simulink model "Pointing_Cntrl_Act"  (R2013a)
settings: Solver=ode14x  StartTime=0.0  StopTime=500  FixedStep=0.01  RelTol=1e-3
values from neighbouring files (symbols this model uses):
  J1 = 4.2946e-2    (= 0.042946)    [RUNCODE_Pointing_CntrlACT.m]    (also in Satellite_Plant_Model.m = 0.000777537)
  J2 = 5.7648e-2    (= 0.057648)    [RUNCODE_Pointing_CntrlACT.m]    (also in Satellite_Plant_Model.m = 8.06522e-05)
  J3 = 1.9229e-2    (= 0.019229)    [RUNCODE_Pointing_CntrlACT.m]    (also in Satellite_Plant_Model.m = 0.0003439929)
  kq = 1    [Control_Block.m]    (also in RUNCODE_Pointing_CntrlACT.m)
  kw = 1    [Control_Block.m]    (also in RUNCODE_Pointing_CntrlACT.m)
  omega1_IC = 0    [RUNCODE_Pointing_CntrlACT.m]
  omega2_IC = 0    [RUNCODE_Pointing_CntrlACT.m]
  omega3_IC = 0    [RUNCODE_Pointing_CntrlACT.m]
  phi_des = 30    [RUNCODE_Pointing_CntrlACT.m]
  phi_dot_des = 0    [RUNCODE_Pointing_CntrlACT.m]
  psi_des = 90    [RUNCODE_Pointing_CntrlACT.m]
  psi_dot_des = 0    [RUNCODE_Pointing_CntrlACT.m]
  q1_IC = 0.1    [RUNCODE_Pointing_CntrlACT.m]
  q2_IC = 0.2    [RUNCODE_Pointing_CntrlACT.m]
  q3_IC = 0.3    [RUNCODE_Pointing_CntrlACT.m]
  q4_IC = 0.92736    [RUNCODE_Pointing_CntrlACT.m]
  theta_des = 120    [RUNCODE_Pointing_CntrlACT.m]
  theta_dot_des = 0    [RUNCODE_Pointing_CntrlACT.m]
  ts = 0.01    [RUNCODE_Pointing_CntrlACT.m]
libraries: dspmtrx3 x1
settings Model: Creator=Mike  LastModifiedBy=Mike

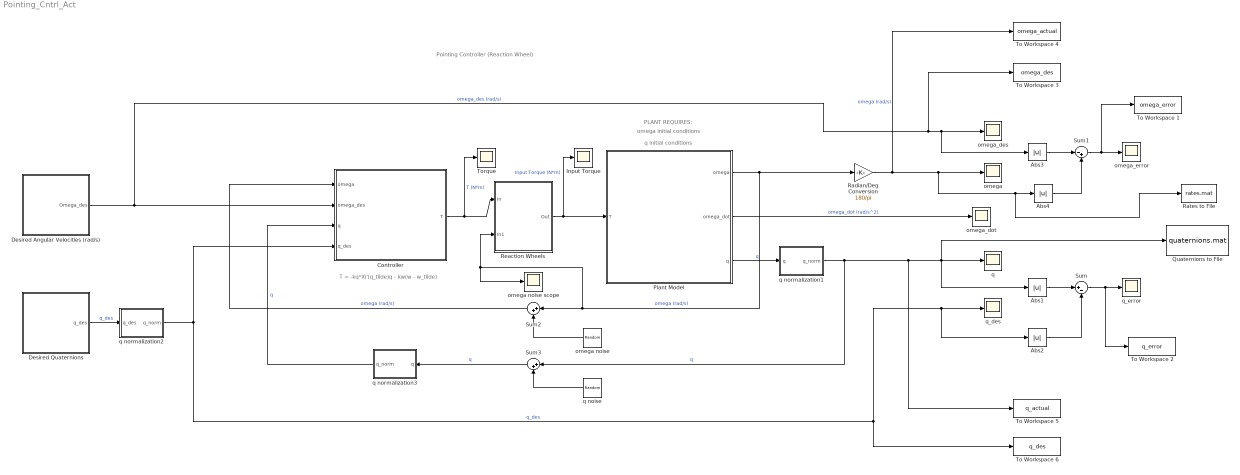
== system Pointing_Cntrl_Act ==
  note: T = -kq*Xi'(q_tilde)q - kw(w - w_tilde)
  note: omega initial conditions
  note: PLANT REQUIRES:
  note: q initial conditions
  note: Pointing Controller (Reaction Wheel)
  " Controller" : Subsystem
  Abs{1..4} (4 alike) : Abs
  Desired Angular Velocities (rad/s) : Subsystem
  Desired Quaternions : Subsystem
  Input Torque : Scope
      settings: TimeRange=500  YMin=-0.0007  YMax=0.0007
  Plant Model : Subsystem
  Quaternions to File : ToFile  Filename=quaternions.mat  MatrixName=quat
  Radian/Deg Conversion : Gain  Gain=180/pi
  Rates to File : ToFile  Filename=rates.mat  MatrixName=omega
  "Reaction Wheels " : Subsystem
  Sum : Sum  Inputs=|+-
  Sum1 : Sum  Inputs=|-+
  Sum2 : Sum  Inputs=|++
  Sum3 : Sum  Inputs=|++
  To Workspace 1 : ToWorkspace  VariableName=omega_error  SampleTime=-1  SaveFormat=Timeseries
  To Workspace 2 : ToWorkspace  VariableName=q_error  SampleTime=-1  SaveFormat=Timeseries
  To Workspace 3 : ToWorkspace  VariableName=omega_des  SampleTime=-1  SaveFormat=Timeseries
  To Workspace 4 : ToWorkspace  VariableName=omega_actual  SampleTime=-1  SaveFormat=Timeseries
  To Workspace 5 : ToWorkspace  VariableName=q_actual  SampleTime=-1  SaveFormat=Timeseries
  To Workspace 6 : ToWorkspace  VariableName=q_des  SampleTime=-1  SaveFormat=Timeseries
  Torque : Scope
      settings: TimeRange=500  YMin=-0.25  YMax=0.275  SaveName=ScopeData5
  omega : Scope
      settings: TimeRange=500  YMin=-15  YMax=10  SaveName=ScopeData3
  omega noise : UniformRandomNumber  Minimum=-.035  Maximum=.035  SampleTime=ts
  omega noise scope : Scope
      settings: TimeRange=500  YMin=-0.55  YMax=0.3  SaveName=ScopeData10
  omega_des : Scope
      settings: YMin=-0.0025  YMax=0.0525  SaveName=ScopeData8
  omega_dot : Scope
      settings: TimeRange=3600  YMin=-0.0004  YMax=-2.5e-05
  omega_error : Scope
      settings: TimeRange=500  YMin=0  YMax=3.25  SaveName=ScopeData7
  q : Scope
      settings: TimeRange=500  YMin=0.225  YMax=0.775  SaveName=ScopeData2
  q noise : UniformRandomNumber  Minimum=-.006  Maximum=.006  SampleTime=ts
  q normalization1 : Subsystem
  q normalization2 : Subsystem
  q normalization3 : Subsystem
  q_des : Scope
      settings: TimeRange=3600  YMin=0.25  YMax=0.75  SaveName=ScopeData4
  q_error : Scope
      settings: TimeRange=3600  YMin=-2e-12  YMax=1e-12  SaveName=ScopeData6
  wires:
  Plant Model/2(omega_dot) -> omega_dot/1  "omega_dot (rad/s^2)"
  " Controller"/1(T) -> "Reaction Wheels "/1(In), Torque/1  "T (N*m)"
  Abs1/1 -> Sum/1
  Abs2/1 -> Sum/2
  Abs3/1 -> Sum1/1
  Abs4/1 -> Sum1/2
  "Reaction Wheels "/1(Out) -> Input Torque/1, Plant Model/1(T)  "Input Torque (N*m)"
  Plant Model/3(q) -> q normalization1/1(q)  "q"
  Desired Quaternions/1(q_des) -> q normalization2/1(q_des)  "q_des"
  Plant Model/1(omega) -> omega noise scope/1, "Reaction Wheels "/2(In1), Sum2/1, Radian/Deg Conversion/1  "omega (rad/s)"
  Sum3/1 -> q normalization3/1(q)  "q"
  q normalization3/1(q_norm) -> " Controller"/3(q)  "q"
  Sum2/1 -> " Controller"/1(omega)  "omega (rad/s)"
  omega noise/1 -> Sum2/2
  q noise/1 -> Sum3/2
  Radian/Deg Conversion/1 -> omega/1, Rates to File/1, Abs4/1, To Workspace 4/1  "omega (rad/s)"
  Desired Angular Velocities (rad/s)/1(Omega_des) -> " Controller"/2(omega_des), To Workspace 3/1, omega_des/1, Abs3/1  "omega_des (rad/s)"
  Sum1/1 -> To Workspace 1/1, omega_error/1
  Sum/1 -> To Workspace 2/1, q_error/1
  q normalization1/1(q_norm) -> Sum3/1, To Workspace 5/1, Quaternions to File/1, Abs1/1, q/1  "q"
  q normalization2/1(q_norm) -> To Workspace 6/1, Abs2/1, q_des/1, " Controller"/4(q_des)  "q_des"

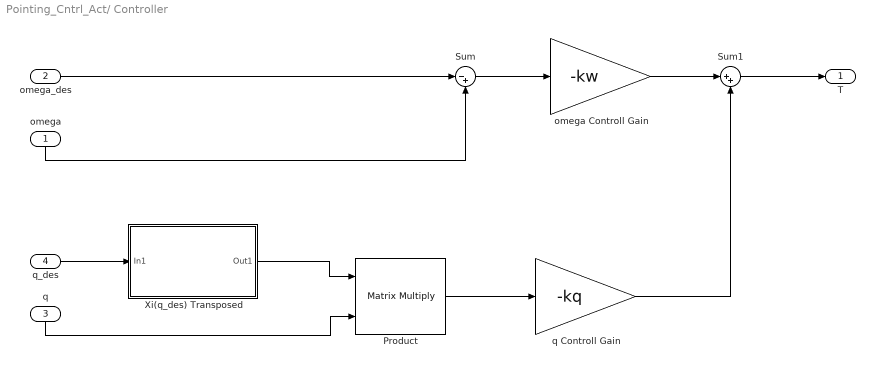
== system Pointing_Cntrl_Act/ Controller ==
  omega : Inport
  omega_des : Inport  Port=2
  q : Inport  Port=3
  q_des : Inport  Port=4
  Product : Product  Multiplication=Matrix(*)
  Sum : Sum  Inputs=|-+
  Sum1 : Sum  Inputs=|++
  Xi(q_des) Transposed : Subsystem
  omega Controll Gain : Gain  Gain=-kw
  q Controll Gain : Gain  Gain=-kq
  T : Outport
  wires:
  q_des/1 -> Xi(q_des) Transposed/1(In1)
  omega_des/1 -> Sum/1
  omega/1 -> Sum/2
  q/1 -> Product/2
  omega Controll Gain/1 -> Sum1/1
  Sum1/1 -> T/1
  Sum/1 -> omega Controll Gain/1
  Xi(q_des) Transposed/1(Out1) -> Product/1
  Product/1 -> q Controll Gain/1
  q Controll Gain/1 -> Sum1/2

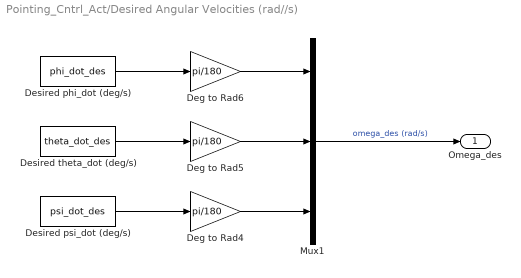
== system Pointing_Cntrl_Act/Desired Angular Velocities (rad//s) ==
  Deg to Rad4 : Gain  Gain=pi/180
  Deg to Rad5 : Gain  Gain=pi/180
  Deg to Rad6 : Gain  Gain=pi/180
  Desired phi_dot (deg/s) : Constant  Value=phi_dot_des
  Desired psi_dot (deg/s) : Constant  Value=psi_dot_des
  Desired theta_dot (deg/s) : Constant  Value=theta_dot_des
  Mux1 : Mux  Inputs=3
  Omega_des : Outport
  wires:
  Mux1/1 -> Omega_des/1  "omega_des (rad/s)"
  Deg to Rad4/1 -> Mux1/3
  Desired theta_dot (deg/s)/1 -> Deg to Rad5/1
  Desired psi_dot (deg/s)/1 -> Deg to Rad4/1
  Desired phi_dot (deg/s)/1 -> Deg to Rad6/1
  Deg to Rad6/1 -> Mux1/1
  Deg to Rad5/1 -> Mux1/2

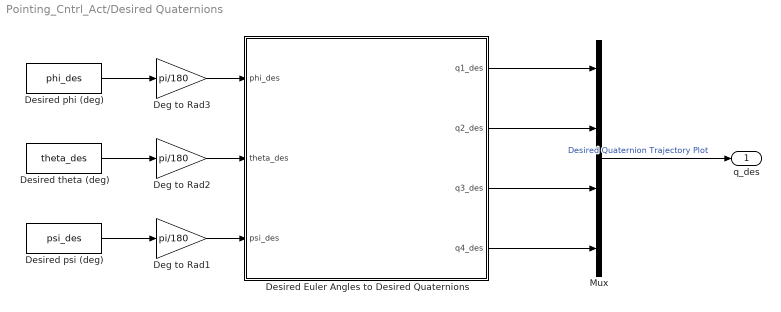
== system Pointing_Cntrl_Act/Desired Quaternions ==
  Deg to Rad1 : Gain  Gain=pi/180
  Deg to Rad2 : Gain  Gain=pi/180
  Deg to Rad3 : Gain  Gain=pi/180
  Desired Euler Angles to Desired Quaternions : MATLAB Function  TreatAsAtomicUnit=on
  Desired phi (deg) : Constant  Value=phi_des
  Desired psi (deg) : Constant  Value=psi_des
  Desired theta (deg) : Constant  Value=theta_des
  Mux : Mux
  q_des : Outport
  wires:
  Mux/1 -> q_des/1  "Desired Quaternion Trajectory Plot"
  Desired theta (deg)/1 -> Deg to Rad2/1
  Deg to Rad3/1 -> Desired Euler Angles to Desired Quaternions/1(phi_des)
  Desired Euler Angles to Desired Quaternions/2(q2_des) -> Mux/2
  Desired Euler Angles to Desired Quaternions/1(q1_des) -> Mux/1
  Deg to Rad1/1 -> Desired Euler Angles to Desired Quaternions/3(psi_des)
  Desired phi (deg)/1 -> Deg to Rad3/1
  Desired psi (deg)/1 -> Deg to Rad1/1
  Deg to Rad2/1 -> Desired Euler Angles to Desired Quaternions/2(theta_des)
  Desired Euler Angles to Desired Quaternions/3(q3_des) -> Mux/3
  Desired Euler Angles to Desired Quaternions/4(q4_des) -> Mux/4

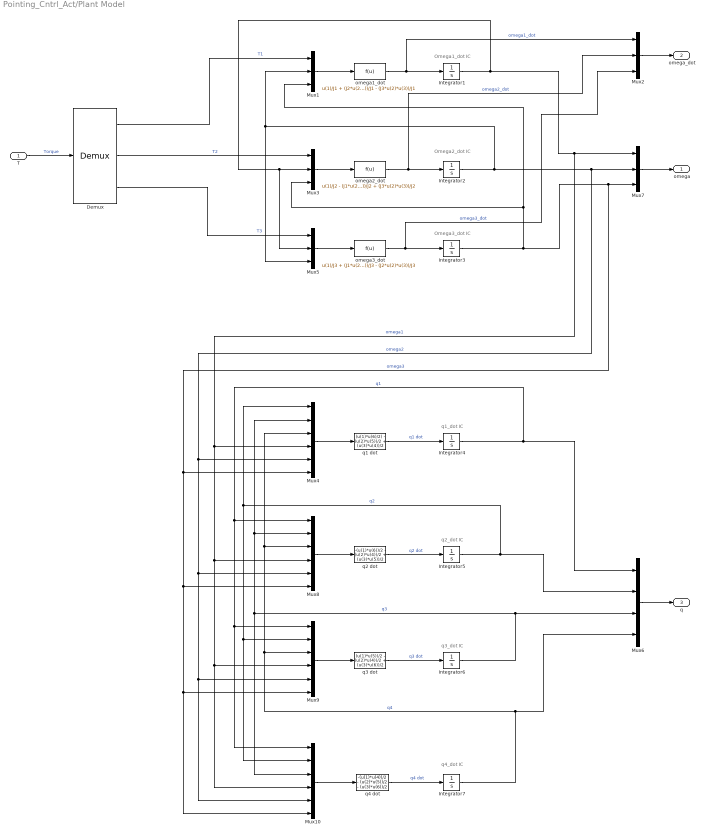
== system Pointing_Cntrl_Act/Plant Model ==
  note: Omega1_dot IC
  note: Omega2_dot IC
  note: Omega3_dot IC
  note: q1_dot IC
  note: q2_dot IC
  note: q3_dot IC
  note: q4_dot IC
  T : Inport
  Demux : Demux  Outputs=3
  Integrator1 : Integrator  InitialCondition=omega1_IC  AbsoluteTolerance=1e-3  ContinuousStateAttributes='omega1'
  Integrator2 : Integrator  InitialCondition=omega2_IC  AbsoluteTolerance=1e-3  ContinuousStateAttributes='omega2'
  Integrator3 : Integrator  InitialCondition=omega3_IC  AbsoluteTolerance=1e-3  ContinuousStateAttributes='omega3'
  Integrator4 : Integrator  InitialCondition=q1_IC  AbsoluteTolerance=1e-3  ContinuousStateAttributes='omega1'
  Integrator5 : Integrator  InitialCondition=q2_IC  AbsoluteTolerance=1e-3  ContinuousStateAttributes='omega1'
  Integrator6 : Integrator  InitialCondition=q3_IC  AbsoluteTolerance=1e-3  ContinuousStateAttributes='omega1'
  Integrator7 : Integrator  InitialCondition=q4_IC  AbsoluteTolerance=1e-3  ContinuousStateAttributes='omega1'
  Mux{1..3,5,7} (5 alike) : Mux  Inputs=3
  Mux{4,8..10} (4 alike) : Mux  Inputs=6
  Mux6 : Mux
  omega1_dot : Fcn  Expr=u(1)/J1 + (J2*u(2)*u(3))/J1 - (J3*u(2)*u(3))/J1
  omega2_dot : Fcn  Expr=u(1)/J2 - (J1*u(2)*u(3))/J2 + (J3*u(2)*u(3))/J2
  omega3_dot : Fcn  Expr=u(1)/J3 + (J1*u(2)*u(3))/J3 - (J2*u(2)*u(3))/J3
  q1 dot : Fcn  Expr=(u(1)*u(6)/2) - (u(2)*u(5))/2 + (u(3)*u(4))/2
  q2 dot : Fcn  Expr=-(u(1)*u(6))/2 - (u(2)*u(4))/2 + (u(3)*u(5))/2
  q3 dot : Fcn  Expr=(u(1)*u(5))/2 - (u(2)*u(4))/2 + (u(3)*u(6))/2
  q4 dot : Fcn  Expr=-(u(1)*u(4))/2 - (u(2)*u(5))/2 - (u(3)*u(6))/2
  omega : Outport
  omega_dot : Outport  Port=2
  q : Outport  Port=3
  wires:
  Demux/3 -> Mux5/1  "T3"
  T/1 -> Demux/1  "Torque"
  Mux7/1 -> omega/1
  Mux1/1 -> omega1_dot/1
  Integrator5/1 -> Mux9/2, Mux10/2, Mux4/1, Mux6/2  "q2"
  q3 dot/1 -> Integrator6/1  "q3 dot"
  Integrator6/1 -> Mux10/3, Mux8/2, Mux4/2, Mux6/3  "q3"
  Integrator7/1 -> Mux6/4, Mux9/3, Mux8/3, Mux4/3  "q4"
  omega3_dot/1 -> Mux2/3, Integrator3/1  "omega3_dot"
  Mux4/1 -> q1 dot/1
  omega2_dot/1 -> Mux2/2, Integrator2/1  "omega2_dot"
  q4 dot/1 -> Integrator7/1  "q4 dot"
  omega1_dot/1 -> Integrator1/1, Mux2/1  "omega1_dot"
  Mux5/1 -> omega3_dot/1
  q1 dot/1 -> Integrator4/1  "q1 dot"
  Mux8/1 -> q2 dot/1
  Integrator1/1 -> Mux7/1, Mux4/4, Mux8/4, Mux10/4, Mux9/4, Mux3/2, Mux5/2  "omega1"
  Integrator2/1 -> Mux7/2, Mux4/5, Mux8/5, Mux10/5, Mux9/5, Mux5/3, Mux1/2  "omega2"
  q2 dot/1 -> Integrator5/1  "q2 dot"
  Mux10/1 -> q4 dot/1
  Mux9/1 -> q3 dot/1
  Mux6/1 -> q/1
  Integrator4/1 -> Mux8/1, Mux9/1, Mux10/1, Mux6/1  "q1"
  Integrator3/1 -> Mux3/3, Mux1/3, Mux7/3, Mux4/6, Mux10/6, Mux9/6, Mux8/6  "omega3"
  Mux3/1 -> omega2_dot/1
  Demux/2 -> Mux3/1  "T2"
  Demux/1 -> Mux1/1  "T1"
  Mux2/1 -> omega_dot/1

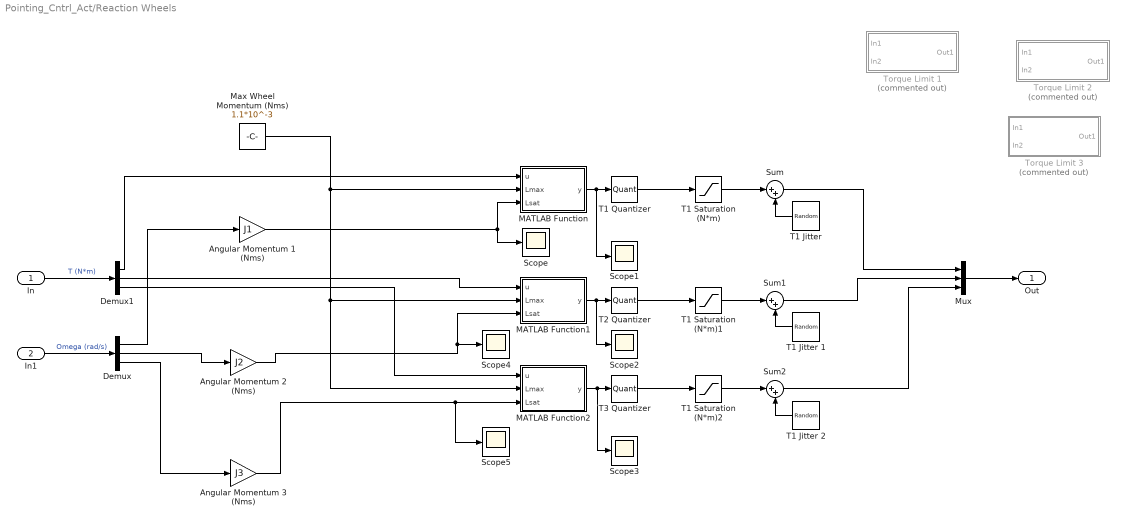
== system Pointing_Cntrl_Act/Reaction Wheels  ==
  In : Inport
  In1 : Inport  Port=2
  "Angular Momentum 1 (Nms) " : Gain  Gain=J1
  Angular Momentum 2 (Nms) : Gain  Gain=J2
  Angular Momentum 3 (Nms) : Gain  Gain=J3
  Demux : Demux  Outputs=3
  Demux1 : Demux  Outputs=3
  MATLAB Function : MATLAB Function  TreatAsAtomicUnit=on
  MATLAB Function1 : MATLAB Function  TreatAsAtomicUnit=on
  MATLAB Function2 : MATLAB Function  TreatAsAtomicUnit=on
  "Max Wheel Momentum (Nms) " : Constant  Value=1.1*10^-3
  Mux : Mux  Inputs=3
  Scope{,1..5} (6 alike) : Scope
      Scope settings: YMin=-0.0075  YMax=0.0175  SaveName=ScopeData11
      Scope1 settings: YMin=-7.5  YMax=0.5  SaveName=ScopeData12
      Scope2 settings: YMin=-0.0075  YMax=0.0175  SaveName=ScopeData13
      Scope3 settings: YMin=-0.0075  YMax=0.0175  SaveName=ScopeData14
      Scope4 settings: YMin=-0.0075  YMax=0.0175  SaveName=ScopeData15
      Scope5 settings: YMin=-0.0005  YMax=0.0005  SaveName=ScopeData16
  Sum : Sum  Inputs=|++
  Sum1 : Sum  Inputs=|++
  Sum2 : Sum  Inputs=|++
  "T1 Jitter " : UniformRandomNumber  Minimum=-0.0005*10^-3  Maximum=0.0005*10^-3  SampleTime=ts
  T1 Jitter 1 : UniformRandomNumber  Minimum=-0.0005*10^-3  Maximum=0.001*10^-3  SampleTime=ts
  T1 Jitter 2 : UniformRandomNumber  Minimum=-0.0005*10^-3  Maximum=0.001*10^-3  SampleTime=ts
  T1 Quantizer : Quantizer  QuantizationInterval=0.02*10^-3
  T1 Saturation (N*m) : Saturate  UpperLimit=0.635/1000  LowerLimit=-0.635/1000
  T1 Saturation (N*m)1 : Saturate  UpperLimit=0.635/1000  LowerLimit=-0.635/1000
  T1 Saturation (N*m)2 : Saturate  UpperLimit=0.635/1000  LowerLimit=-0.635/1000
  T2 Quantizer : Quantizer  QuantizationInterval=0.02*10^-3
  T3 Quantizer : Quantizer  QuantizationInterval=0.02*10^-3
  Torque Limit 1 : Subsystem  Commented=on  TreatAsAtomicUnit=on
  Torque Limit 2 : Subsystem  Commented=on  TreatAsAtomicUnit=on
  Torque Limit 3 : Subsystem  Commented=on  TreatAsAtomicUnit=on
  Out : Outport
  wires:
  In/1 -> Demux1/1  "T (N*m)"
  Demux1/2 -> MATLAB Function1/1(u)
  Demux1/1 -> MATLAB Function/1(u)
  Mux/1 -> Out/1
  In1/1 -> Demux/1  "Omega (rad/s)"
  Demux/1 -> "Angular Momentum 1 (Nms) "/1
  Demux/2 -> Angular Momentum 2 (Nms)/1
  Demux/3 -> Angular Momentum 3 (Nms)/1
  "Max Wheel Momentum (Nms) "/1 -> MATLAB Function/2(Lmax), MATLAB Function2/2(Lmax), MATLAB Function1/2(Lmax)
  Angular Momentum 2 (Nms)/1 -> Scope4/1, MATLAB Function1/3(Lsat)
  Angular Momentum 3 (Nms)/1 -> Scope5/1, MATLAB Function2/3(Lsat)
  T1 Quantizer/1 -> T1 Saturation (N*m)/1
  MATLAB Function/1(y) -> Scope1/1, T1 Quantizer/1
  T1 Saturation (N*m)/1 -> Sum/1
  Sum/1 -> Mux/1
  "T1 Jitter "/1 -> Sum/2
  MATLAB Function1/1(y) -> Scope2/1, T2 Quantizer/1
  T1 Saturation (N*m)1/1 -> Sum1/1
  T1 Jitter 1/1 -> Sum1/2
  T2 Quantizer/1 -> T1 Saturation (N*m)1/1
  Sum1/1 -> Mux/2
  T1 Saturation (N*m)2/1 -> Sum2/1
  T1 Jitter 2/1 -> Sum2/2
  T3 Quantizer/1 -> T1 Saturation (N*m)2/1
  Sum2/1 -> Mux/3
  MATLAB Function2/1(y) -> Scope3/1, T3 Quantizer/1
  Demux1/3 -> MATLAB Function2/1(u)
  "Angular Momentum 1 (Nms) "/1 -> MATLAB Function/3(Lsat), Scope/1

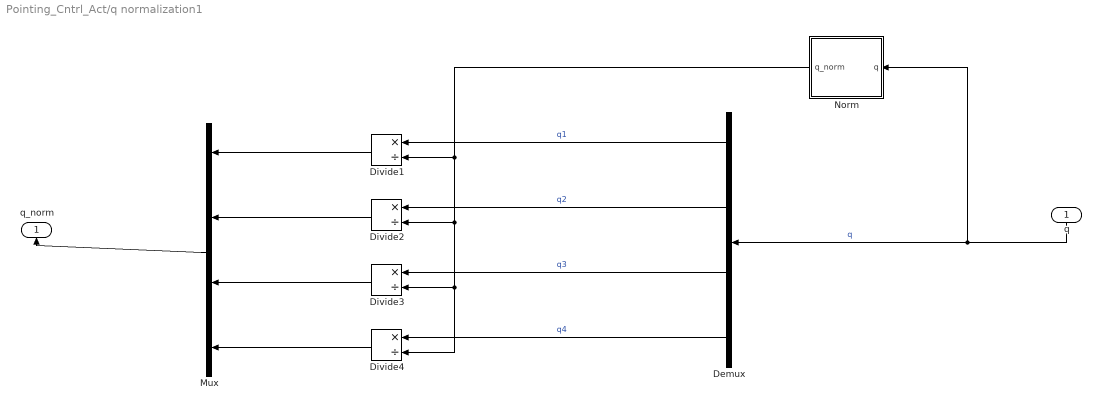
== system Pointing_Cntrl_Act/q normalization1 ==
  q : Inport
  Demux : Demux
  Divide{1..4} (4 alike) : Product  Inputs=*/
  Mux : Mux
  Norm : MATLAB Function  TreatAsAtomicUnit=on
  q_norm : Outport
  wires:
  Divide1/1 -> Mux/1
  Divide2/1 -> Mux/2
  Divide3/1 -> Mux/3
  Divide4/1 -> Mux/4
  Mux/1 -> q_norm/1
  Demux/2 -> Divide2/1  "q2"
  Demux/3 -> Divide3/1  "q3"
  Demux/4 -> Divide4/1  "q4"
  Demux/1 -> Divide1/1  "q1"
  Norm/1(q_norm) -> Divide1/2, Divide2/2, Divide3/2, Divide4/2
  q/1 -> Norm/1(q), Demux/1  "q"

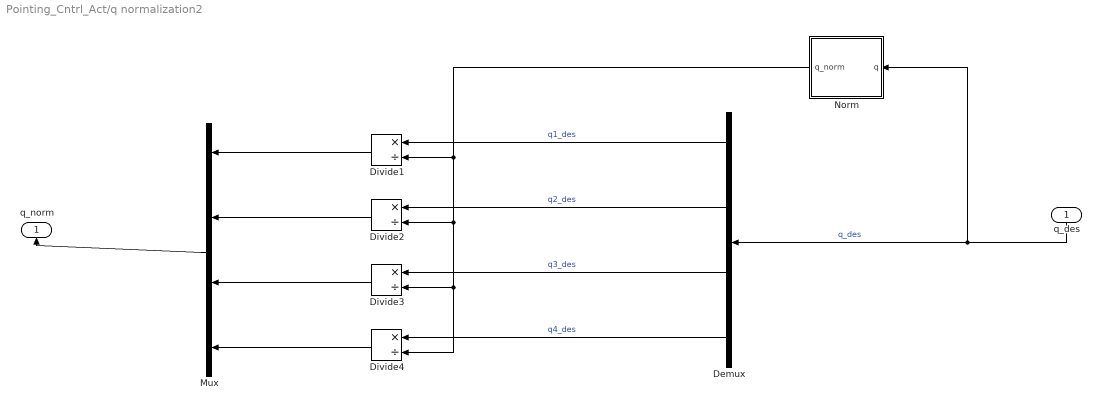
== system Pointing_Cntrl_Act/q normalization2 ==
  q_des : Inport
  Demux : Demux
  Divide{1..4} (4 alike) : Product  Inputs=*/
  Mux : Mux
  Norm : MATLAB Function  TreatAsAtomicUnit=on
  q_norm : Outport
  wires:
  Divide1/1 -> Mux/1
  Divide2/1 -> Mux/2
  Divide3/1 -> Mux/3
  Divide4/1 -> Mux/4
  Mux/1 -> q_norm/1
  Demux/2 -> Divide2/1  "q2_des"
  Demux/3 -> Divide3/1  "q3_des"
  Demux/4 -> Divide4/1  "q4_des"
  Demux/1 -> Divide1/1  "q1_des"
  Norm/1(q_norm) -> Divide1/2, Divide2/2, Divide3/2, Divide4/2
  q_des/1 -> Norm/1(q), Demux/1  "q_des"

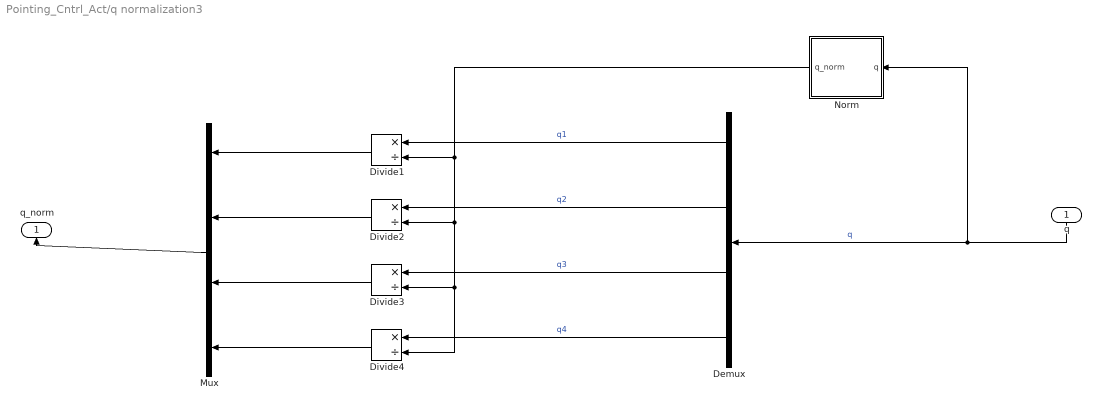
== system Pointing_Cntrl_Act/q normalization3 ==
  q : Inport
  Demux : Demux
  Divide{1..4} (4 alike) : Product  Inputs=*/
  Mux : Mux
  Norm : MATLAB Function  TreatAsAtomicUnit=on
  q_norm : Outport
  wires:
  Divide1/1 -> Mux/1
  Divide2/1 -> Mux/2
  Divide3/1 -> Mux/3
  Divide4/1 -> Mux/4
  Mux/1 -> q_norm/1
  Demux/2 -> Divide2/1  "q2"
  Demux/3 -> Divide3/1  "q3"
  Demux/4 -> Divide4/1  "q4"
  Demux/1 -> Divide1/1  "q1"
  Norm/1(q_norm) -> Divide1/2, Divide2/2, Divide3/2, Divide4/2
  q/1 -> Norm/1(q), Demux/1  "q"

== system Pointing_Cntrl_Act/ Controller/Xi(q_des) Transposed ==
  In1 : Inport
  Demux : Demux
  Transpose : dspmtrx3/Transpose  Hermitian=off  overflowFlag=off
  Xi_qtilde = Xi(q_des) : MATLAB Function  TreatAsAtomicUnit=on
  Out1 : Outport
  wires:
  In1/1 -> Demux/1
  Demux/4 -> Xi_qtilde = Xi(q_des)/4(q4_des)
  Demux/2 -> Xi_qtilde = Xi(q_des)/2(q2_des)
  Demux/1 -> Xi_qtilde = Xi(q_des)/1(q1_des)
  Transpose/1 -> Out1/1
  Xi_qtilde = Xi(q_des)/1(Xi_qtilde) -> Transpose/1
  Demux/3 -> Xi_qtilde = Xi(q_des)/3(q3_des)

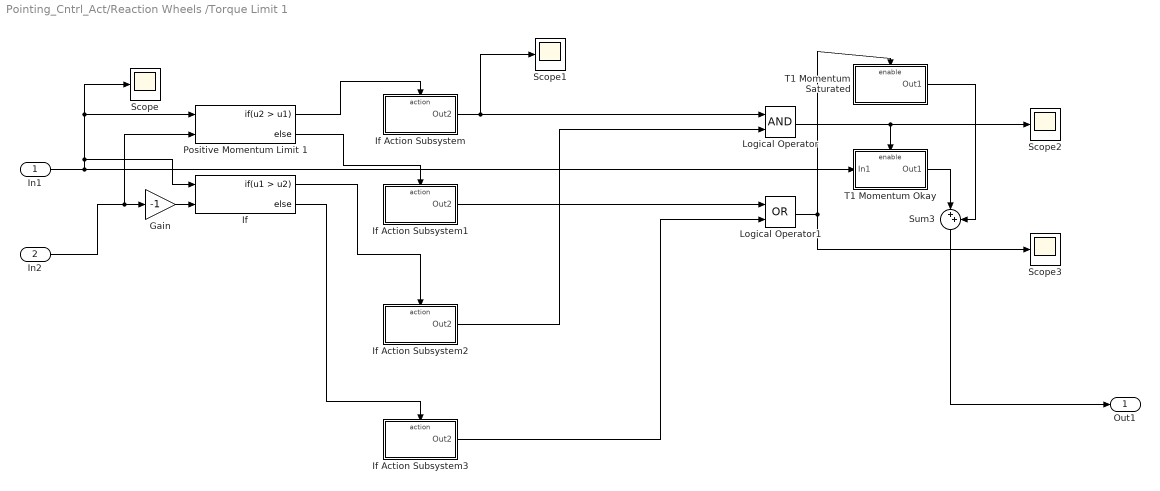
== system Pointing_Cntrl_Act/Reaction Wheels /Torque Limit 1 ==
  In1 : Inport
  In2 : Inport  Port=2
  Gain : Gain  Gain=-1
  If : If  NumInputs=2  IfExpression=u1 > u2
  If Action Subsystem : Subsystem  TreatAsAtomicUnit=on
  If Action Subsystem1 : Subsystem  TreatAsAtomicUnit=on
  If Action Subsystem2 : Subsystem  TreatAsAtomicUnit=on
  If Action Subsystem3 : Subsystem  TreatAsAtomicUnit=on
  Logical Operator : Logic  AllPortsSameDT=off  OutDataTypeStr=boolean
  Logical Operator1 : Logic  Operator=OR  AllPortsSameDT=off  OutDataTypeStr=boolean
  Positive Momentum Limit 1 : If  NumInputs=2  IfExpression=u2 > u1
  Scope{,1..3} (4 alike) : Scope
      Scope settings: YMin=-1.5  YMax=8  SaveName=ScopeData17
      Scope1 settings: YMin=-1.5  YMax=8  SaveName=ScopeData18
      Scope2 settings: YMin=-1.5  YMax=8  SaveName=ScopeData19
      Scope3 settings: YMin=-1.5  YMax=8  SaveName=ScopeData20
  Sum3 : Sum  Inputs=|++
  T1 Momentum Okay : Subsystem  TreatAsAtomicUnit=on
  "T1 Momentum Saturated " : Subsystem  TreatAsAtomicUnit=on
  Out1 : Outport
  wires:
  In1/1 -> T1 Momentum Okay/1(In1), Scope/1, Positive Momentum Limit 1/1, If/1
  In2/1 -> Positive Momentum Limit 1/2, Gain/1
  T1 Momentum Okay/1(Out1) -> Sum3/1
  Sum3/1 -> Out1/1
  "T1 Momentum Saturated "/1(Out1) -> Sum3/2
  Gain/1 -> If/2
  Logical Operator/1 -> Scope2/1, T1 Momentum Okay/Enable
  Logical Operator1/1 -> "T1 Momentum Saturated "/Enable, Scope3/1
  Positive Momentum Limit 1/1 -> If Action Subsystem/Action
  If/2 -> If Action Subsystem3/Action
  Positive Momentum Limit 1/2 -> If Action Subsystem1/Action
  If/1 -> If Action Subsystem2/Action
  If Action Subsystem/1(Out2) -> Scope1/1, Logical Operator/1
  If Action Subsystem2/1(Out2) -> Logical Operator/2
  If Action Subsystem1/1(Out2) -> Logical Operator1/1
  If Action Subsystem3/1(Out2) -> Logical Operator1/2

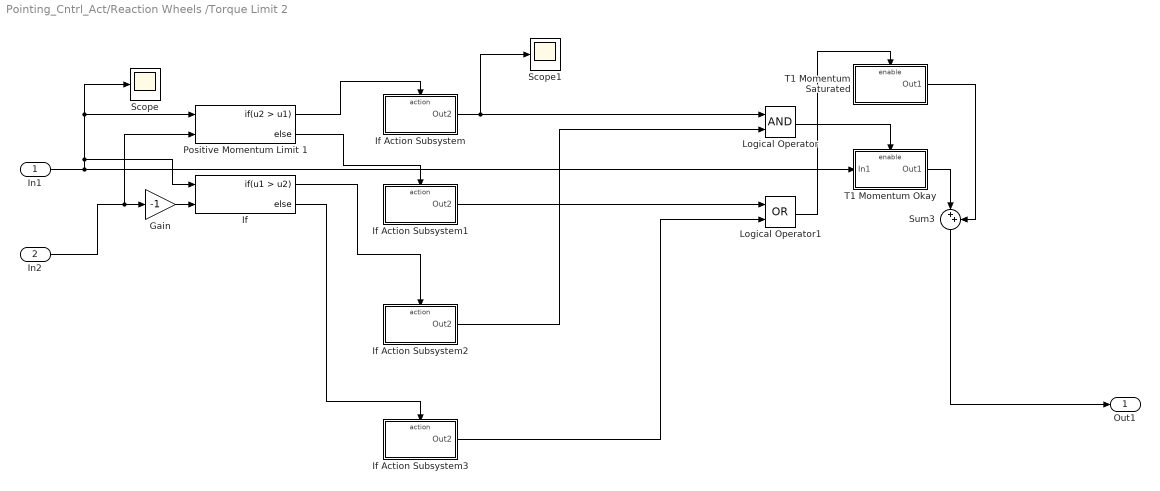
== system Pointing_Cntrl_Act/Reaction Wheels /Torque Limit 2 ==
  In1 : Inport
  In2 : Inport  Port=2
  Gain : Gain  Gain=-1
  If : If  NumInputs=2  IfExpression=u1 > u2
  If Action Subsystem : Subsystem  TreatAsAtomicUnit=on
  If Action Subsystem1 : Subsystem  TreatAsAtomicUnit=on
  If Action Subsystem2 : Subsystem  TreatAsAtomicUnit=on
  If Action Subsystem3 : Subsystem  TreatAsAtomicUnit=on
  Logical Operator : Logic  AllPortsSameDT=off  OutDataTypeStr=boolean
  Logical Operator1 : Logic  Operator=OR  AllPortsSameDT=off  OutDataTypeStr=boolean
  Positive Momentum Limit 1 : If  NumInputs=2  IfExpression=u2 > u1
  Scope : Scope
      settings: YMin=-1.5  YMax=8  SaveName=ScopeData17
  Scope1 : Scope
      settings: YMin=-1.5  YMax=8  SaveName=ScopeData18
  Sum3 : Sum  Inputs=|++
  T1 Momentum Okay : Subsystem  TreatAsAtomicUnit=on
  "T1 Momentum Saturated " : Subsystem  TreatAsAtomicUnit=on
  Out1 : Outport
  wires:
  In1/1 -> T1 Momentum Okay/1(In1), Scope/1, Positive Momentum Limit 1/1, If/1
  In2/1 -> Positive Momentum Limit 1/2, Gain/1
  T1 Momentum Okay/1(Out1) -> Sum3/1
  Sum3/1 -> Out1/1
  "T1 Momentum Saturated "/1(Out1) -> Sum3/2
  Gain/1 -> If/2
  Logical Operator/1 -> T1 Momentum Okay/Enable
  Logical Operator1/1 -> "T1 Momentum Saturated "/Enable
  Positive Momentum Limit 1/1 -> If Action Subsystem/Action
  If/2 -> If Action Subsystem3/Action
  Positive Momentum Limit 1/2 -> If Action Subsystem1/Action
  If/1 -> If Action Subsystem2/Action
  If Action Subsystem/1(Out2) -> Scope1/1, Logical Operator/1
  If Action Subsystem2/1(Out2) -> Logical Operator/2
  If Action Subsystem1/1(Out2) -> Logical Operator1/1
  If Action Subsystem3/1(Out2) -> Logical Operator1/2

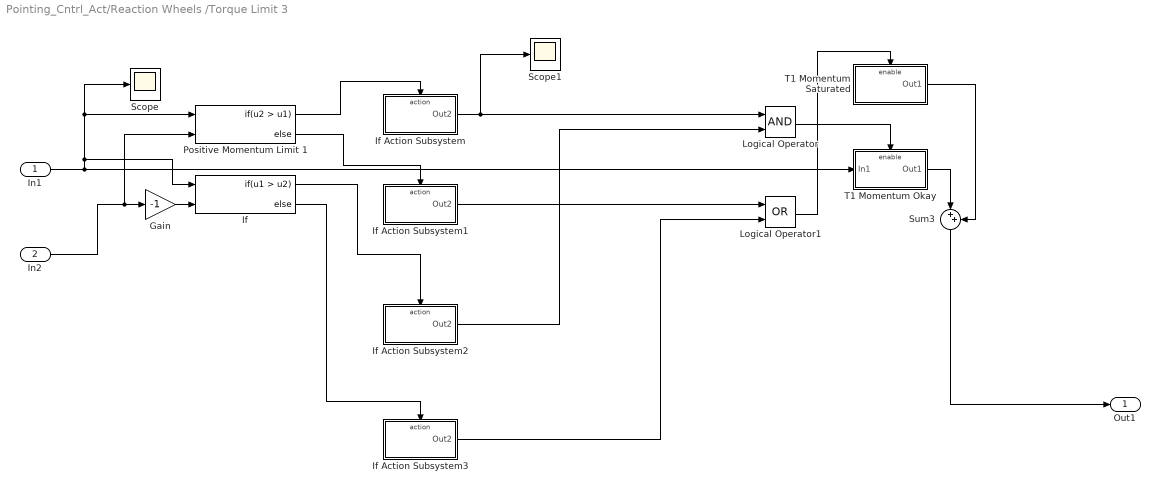
== system Pointing_Cntrl_Act/Reaction Wheels /Torque Limit 3 ==
  In1 : Inport
  In2 : Inport  Port=2
  Gain : Gain  Gain=-1
  If : If  NumInputs=2  IfExpression=u1 > u2
  If Action Subsystem : Subsystem  TreatAsAtomicUnit=on
  If Action Subsystem1 : Subsystem  TreatAsAtomicUnit=on
  If Action Subsystem2 : Subsystem  TreatAsAtomicUnit=on
  If Action Subsystem3 : Subsystem  TreatAsAtomicUnit=on
  Logical Operator : Logic  AllPortsSameDT=off  OutDataTypeStr=boolean
  Logical Operator1 : Logic  Operator=OR  AllPortsSameDT=off  OutDataTypeStr=boolean
  Positive Momentum Limit 1 : If  NumInputs=2  IfExpression=u2 > u1
  Scope : Scope
      settings: YMin=-1.5  YMax=8  SaveName=ScopeData17
  Scope1 : Scope
      settings: YMin=-1.5  YMax=8  SaveName=ScopeData18
  Sum3 : Sum  Inputs=|++
  T1 Momentum Okay : Subsystem  TreatAsAtomicUnit=on
  "T1 Momentum Saturated " : Subsystem  TreatAsAtomicUnit=on
  Out1 : Outport
  wires:
  In1/1 -> T1 Momentum Okay/1(In1), Scope/1, Positive Momentum Limit 1/1, If/1
  In2/1 -> Positive Momentum Limit 1/2, Gain/1
  T1 Momentum Okay/1(Out1) -> Sum3/1
  Sum3/1 -> Out1/1
  "T1 Momentum Saturated "/1(Out1) -> Sum3/2
  Gain/1 -> If/2
  Logical Operator/1 -> T1 Momentum Okay/Enable
  Logical Operator1/1 -> "T1 Momentum Saturated "/Enable
  Positive Momentum Limit 1/1 -> If Action Subsystem/Action
  If/2 -> If Action Subsystem3/Action
  Positive Momentum Limit 1/2 -> If Action Subsystem1/Action
  If/1 -> If Action Subsystem2/Action
  If Action Subsystem/1(Out2) -> Scope1/1, Logical Operator/1
  If Action Subsystem2/1(Out2) -> Logical Operator/2
  If Action Subsystem1/1(Out2) -> Logical Operator1/1
  If Action Subsystem3/1(Out2) -> Logical Operator1/2

== system Pointing_Cntrl_Act/Reaction Wheels /Torque Limit 1/If Action Subsystem ==
  Action Port : ActionPort  InitializeStates=reset
  Constant : Constant  Value=true  OutDataTypeStr=boolean
  Out2 : Outport  OutDataTypeStr=boolean  OutputWhenDisabled=reset  InitialOutput=[false]
  wires:
  Constant/1 -> Out2/1

== system Pointing_Cntrl_Act/Reaction Wheels /Torque Limit 1/If Action Subsystem1 ==
  Action Port : ActionPort  InitializeStates=reset
  Constant : Constant  Value=true  OutDataTypeStr=boolean
  Out2 : Outport  OutDataTypeStr=boolean  OutputWhenDisabled=reset  InitialOutput=[false]
  wires:
  Constant/1 -> Out2/1

== system Pointing_Cntrl_Act/Reaction Wheels /Torque Limit 1/If Action Subsystem2 ==
  Action Port : ActionPort  InitializeStates=reset
  Constant : Constant  Value=true  OutDataTypeStr=boolean
  Out2 : Outport  OutDataTypeStr=boolean  OutputWhenDisabled=reset  InitialOutput=[false]
  wires:
  Constant/1 -> Out2/1

== system Pointing_Cntrl_Act/Reaction Wheels /Torque Limit 1/If Action Subsystem3 ==
  Action Port : ActionPort  InitializeStates=reset
  Constant : Constant  Value=true  OutDataTypeStr=boolean
  Out2 : Outport  OutDataTypeStr=boolean  OutputWhenDisabled=reset  InitialOutput=[false]
  wires:
  Constant/1 -> Out2/1

== system Pointing_Cntrl_Act/Reaction Wheels /Torque Limit 1/T1 Momentum Okay ==
  In1 : Inport
  Enable : EnablePort  StatesWhenEnabling=reset
  Sum : Sum  Inputs=|++
  "T1 Jitter " : UniformRandomNumber  Minimum=-0.005  Maximum=0.005  SampleTime=ts
  T1 Saturation (N*m) : Saturate  UpperLimit=0.635/1000  LowerLimit=-0.635/1000
  Out1 : Outport  InitialOutput=[0]
  wires:
  T1 Saturation (N*m)/1 -> Sum/1
  "T1 Jitter "/1 -> Sum/2
  Sum/1 -> Out1/1
  In1/1 -> T1 Saturation (N*m)/1

== system Pointing_Cntrl_Act/Reaction Wheels /Torque Limit 1/T1 Momentum Saturated  ==
  Enable : EnablePort  StatesWhenEnabling=reset
  "T1 Jitter " : UniformRandomNumber  Minimum=-0.005  Maximum=0.005  SampleTime=ts
  Out1 : Outport  InitialOutput=[0]
  wires:
  "T1 Jitter "/1 -> Out1/1

== system Pointing_Cntrl_Act/Reaction Wheels /Torque Limit 2/If Action Subsystem ==
  Action Port : ActionPort  InitializeStates=reset
  Constant : Constant  Value=true  OutDataTypeStr=boolean
  Out2 : Outport  OutDataTypeStr=boolean  OutputWhenDisabled=reset  InitialOutput=[false]
  wires:
  Constant/1 -> Out2/1

== system Pointing_Cntrl_Act/Reaction Wheels /Torque Limit 2/If Action Subsystem1 ==
  Action Port : ActionPort  InitializeStates=reset
  Constant : Constant  Value=true  OutDataTypeStr=boolean
  Out2 : Outport  OutDataTypeStr=boolean  OutputWhenDisabled=reset  InitialOutput=[false]
  wires:
  Constant/1 -> Out2/1

== system Pointing_Cntrl_Act/Reaction Wheels /Torque Limit 2/If Action Subsystem2 ==
  Action Port : ActionPort  InitializeStates=reset
  Constant : Constant  Value=true  OutDataTypeStr=boolean
  Out2 : Outport  OutDataTypeStr=boolean  OutputWhenDisabled=reset  InitialOutput=[false]
  wires:
  Constant/1 -> Out2/1

== system Pointing_Cntrl_Act/Reaction Wheels /Torque Limit 2/If Action Subsystem3 ==
  Action Port : ActionPort  InitializeStates=reset
  Constant : Constant  Value=true  OutDataTypeStr=boolean
  Out2 : Outport  OutDataTypeStr=boolean  OutputWhenDisabled=reset  InitialOutput=[false]
  wires:
  Constant/1 -> Out2/1

== system Pointing_Cntrl_Act/Reaction Wheels /Torque Limit 2/T1 Momentum Okay ==
  In1 : Inport
  Enable : EnablePort  StatesWhenEnabling=reset
  Sum : Sum  Inputs=|++
  "T1 Jitter " : UniformRandomNumber  Minimum=-0.005  Maximum=0.005  SampleTime=ts
  T1 Saturation (N*m) : Saturate  UpperLimit=0.635/1000  LowerLimit=-0.635/1000
  Out1 : Outport  InitialOutput=[0]
  wires:
  T1 Saturation (N*m)/1 -> Sum/1
  "T1 Jitter "/1 -> Sum/2
  Sum/1 -> Out1/1
  In1/1 -> T1 Saturation (N*m)/1

== system Pointing_Cntrl_Act/Reaction Wheels /Torque Limit 2/T1 Momentum Saturated  ==
  Enable : EnablePort  StatesWhenEnabling=reset
  "T1 Jitter " : UniformRandomNumber  Minimum=-0.005  Maximum=0.005  SampleTime=ts
  Out1 : Outport  InitialOutput=[0]
  wires:
  "T1 Jitter "/1 -> Out1/1

== system Pointing_Cntrl_Act/Reaction Wheels /Torque Limit 3/If Action Subsystem ==
  Action Port : ActionPort  InitializeStates=reset
  Constant : Constant  Value=true  OutDataTypeStr=boolean
  Out2 : Outport  OutDataTypeStr=boolean  OutputWhenDisabled=reset  InitialOutput=[false]
  wires:
  Constant/1 -> Out2/1

== system Pointing_Cntrl_Act/Reaction Wheels /Torque Limit 3/If Action Subsystem1 ==
  Action Port : ActionPort  InitializeStates=reset
  Constant : Constant  Value=true  OutDataTypeStr=boolean
  Out2 : Outport  OutDataTypeStr=boolean  OutputWhenDisabled=reset  InitialOutput=[false]
  wires:
  Constant/1 -> Out2/1

== system Pointing_Cntrl_Act/Reaction Wheels /Torque Limit 3/If Action Subsystem2 ==
  Action Port : ActionPort  InitializeStates=reset
  Constant : Constant  Value=true  OutDataTypeStr=boolean
  Out2 : Outport  OutDataTypeStr=boolean  OutputWhenDisabled=reset  InitialOutput=[false]
  wires:
  Constant/1 -> Out2/1

== system Pointing_Cntrl_Act/Reaction Wheels /Torque Limit 3/If Action Subsystem3 ==
  Action Port : ActionPort  InitializeStates=reset
  Constant : Constant  Value=true  OutDataTypeStr=boolean
  Out2 : Outport  OutDataTypeStr=boolean  OutputWhenDisabled=reset  InitialOutput=[false]
  wires:
  Constant/1 -> Out2/1

== system Pointing_Cntrl_Act/Reaction Wheels /Torque Limit 3/T1 Momentum Okay ==
  In1 : Inport
  Enable : EnablePort  StatesWhenEnabling=reset
  Sum : Sum  Inputs=|++
  "T1 Jitter " : UniformRandomNumber  Minimum=-0.005  Maximum=0.005  SampleTime=ts
  T1 Saturation (N*m) : Saturate  UpperLimit=0.635/1000  LowerLimit=-0.635/1000
  Out1 : Outport  InitialOutput=[0]
  wires:
  T1 Saturation (N*m)/1 -> Sum/1
  "T1 Jitter "/1 -> Sum/2
  Sum/1 -> Out1/1
  In1/1 -> T1 Saturation (N*m)/1

== system Pointing_Cntrl_Act/Reaction Wheels /Torque Limit 3/T1 Momentum Saturated  ==
  Enable : EnablePort  StatesWhenEnabling=reset
  "T1 Jitter " : UniformRandomNumber  Minimum=-0.005  Maximum=0.005  SampleTime=ts
  Out1 : Outport  InitialOutput=[0]
  wires:
  "T1 Jitter "/1 -> Out1/1

== matlab function Pointing_Cntrl_Act/Reaction Wheels /MATLAB Function ==
  data: u input; y output; Lmax input; Lsat input
function y = fcn(u,Lmax,Lsat)
%#codegen

if u >= 0
    Llim = Lmax - Lsat;
    if Llim < 0
        y = 0;
    else
        y = min (Llim,u);
    end
else
    Llim = -Lmax - Lsat;
    if Llim > 0
        y = 0;
    else
        y = max(Llim,u);
    end
end

== matlab function Pointing_Cntrl_Act/ Controller/Xi(q_des) Transposed/Xi_qtilde = Xi(q_des) ==
  data: q1_des input; Xi_qtilde output; q2_des input; q3_des input; q4_des input
function Xi_qtilde = fcn(q1_des,q2_des,q3_des,q4_des)
Xi_qtilde=[q4_des  -q3_des   q2_des;
           q3_des   q4_des  -q1_des;
          -q2_des   q1_des   q4_des;
          -q1_des  -q2_des  -q3_des];

== matlab function Pointing_Cntrl_Act/q normalization2/Norm ==
  data: q input; q_norm output
function q_norm = fcn(q)

q_norm = norm(q);

== matlab function Pointing_Cntrl_Act/Reaction Wheels /MATLAB Function1 ==
  data: u input; y output; Lmax input; Lsat input
function y = fcn(u,Lmax,Lsat)
%#codegen

if u >= 0
    Llim = Lmax - Lsat;
    if Llim < 0
        y = 0;
    else
        y = min (Llim,u);
    end
else
    Llim = -Lmax - Lsat;
    if Llim > 0
        y = 0;
    else
        y = max(Llim,u);
    end
end

== matlab function Pointing_Cntrl_Act/q normalization3/Norm ==
  data: q input; q_norm output
function q_norm = fcn(q)

q_norm = norm(q);

== matlab function Pointing_Cntrl_Act/Reaction Wheels /MATLAB Function2 ==
  data: u input; y output; Lmax input; Lsat input
function y = fcn(u,Lmax,Lsat)
%#codegen

if u >= 0
    Llim = Lmax - Lsat;
    if Llim < 0
        y = 0;
    else
        y = min (Llim,u);
    end
else
    Llim = -Lmax - Lsat;
    if Llim > 0
        y = 0;
    else
        y = max(Llim,u);
    end
end

== matlab function Pointing_Cntrl_Act/q normalization1/Norm ==
  data: q input; q_norm output
function q_norm = fcn(q)

q_norm = norm(q);

== matlab function Pointing_Cntrl_Act/Desired Quaternions/Desired Euler Angles to Desired Quaternions ==
  data: phi_des input; q1_des output; q2_des output; q3_des output; q4_des output; theta_des input; psi_des input
function [q1_des,q2_des,q3_des,q4_des]= fcn(phi_des,theta_des,psi_des)
% Desired Euler Angles to Desired Quaternions

    %%  3-1-3 Attitude Matrix Parameters 
    s1 = sin(phi_des);
    s2 = sin(theta_des);
    s3 = sin(psi_des);
    c1 = cos(phi_des);
    c2 = cos(theta_des);
    c3 = cos(psi_des);

    A = [(c1*c3)-(s1*c2*s3), (c1*s3)+(s1*c2*c3), s1*s2;
         (-s1*c3)-(c1*c2*s3), (-s1*s3)+(c1*c2*c3) c1*s2;
          s2*s3,              -s2*c3,             c2;];

    %% Quaternion Parameters 
    q1_des = sqrt((1/4)*(1+A(1,1)-A(2,2)-A(3,3)));
    q2_des = sqrt((1/4)*(1+A(2,2)-A(1,1)-A(3,3)));
    q3_des = sqrt((1/4)*(1+A(3,3)-A(1,1)-A(2,2)));
    q4_des = sqrt((1/4)*(1+A(1,1)+A(2,2)+A(3,3)));
